simulink model "closed12augs"  (R2018b)
settings: Solver=VariableStepAuto  StartTime=0.0  StopTime=1  RelTol=1e-3
libraries: powerlib x63, simulink x5, autolibsharedcoupling x1, simulink_extras x1
settings Model: Creator=Ratish Kumar S  LastModifiedBy=Ratish Kumar S

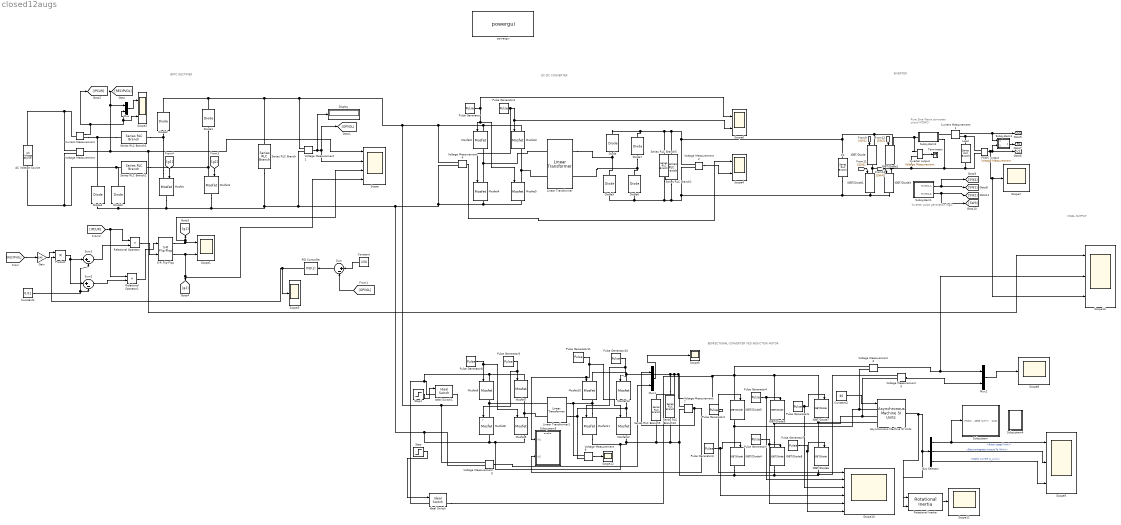
== system closed12augs ==
  note: INVERTER
  note: DC-DC CONVERTER
  note: Inverter pulse generation logic
  note: BPFC RECTIFIER
  note: Pure Sine Wave converter circuit (PSWC)
  note: z
  note: BIDIRECTIONAL CONVERTER FED INDUCTION MOTOR
  note: FINAL OUTPUT
  AC Voltage Source : powerlib/Electrical Sources/AC Voltage Source  Amplitude=230  Phase=0  Frequency=50  SampleTime=0  Measurements=None  BusType=swing  Pref=10e3  Qref=0  Qmin=-inf  Qmax=+inf
      settings: SourceProductName=Simscape Electrical
  Asynchronous Machine SI Units : powerlib/Machines/Asynchronous Machine SI Units  RotorType=Squirrel-cage  PresetModel=No  MechanicalLoad=Torque Tm  ShowDetailedParameters=on  ReferenceFrame=Rotor  Units=SI  MeasurementBus=off  NominalParameters=[1.845e+04 380 50]  Stator=[0.699999 0.00999999]  Rotor=[0.6258 0.005473]  Cage1=[0.4155 0.002066]  Cage2=[0.4168 0.0003495]  Lm=0.0399  Mechanical=[0.05 0.005879 2]  PolePairs=2  InitialConditions=[0 0 0 0 0 0 0 0]  SimulateSaturation=off  Saturation=[14.03593122, 27.81365428, 53.79336849, 72.68890987, 97.98006896, 148.6815601, 215.7428561, 302.9841135, 428.7778367 ; 230, 322, 414, 460, 506, 552, 598, 644, 690]  LoadFlowParameters=1492000  TsPowergui=0  TsBlock=-1  IterativeModel=Trapezoidal non iterative  IterativeDiscreteModel=Trapezoidal non iterative  Pmec=1.492e+006
      settings: SourceProductName=Simscape Electrical
  Bus Selector : BusSelector  OutputSignals=Mechanical.Rotor speed (wm),Mechanical.Electromagnetic torque Te (N*m),Stator measurements.Stator current is_a (A)
  C1 : powerlib/Elements/Series RLC Branch  LConnTagsString=__new0  RConnTagsString=__new0  BranchType=C  Resistance=1  Inductance=1e-3  SetiL0=off  InitialCurrent=0  Capacitance=200e-3  Setx0=off  InitialVoltage=0  Measurements=None
      settings: SourceProductName=Simscape Electrical
  Constant : Constant  Value=230
  Constant1 : Constant  Value=0.01
  Constant2 : Constant  Value=30
  Current Measurement : powerlib/Measurements/Current Measurement  PhasorSimulation=off  OutputType=Complex  PSBequivalent=0
      settings: SourceProductName=Simscape Electrical
  Current Measurement1 : powerlib/Measurements/Current Measurement  PhasorSimulation=off  OutputType=Complex  PSBequivalent=0
      settings: SourceProductName=Simscape Electrical
  Diode{,1..7} (8 alike) : powerlib/Power Electronics/Diode  Ron=0.001  Lon=0  Vf=0.8  IC=0  UseSnubber=off  Rs=500  Cs=250e-9  Measurements=off
      settings: SourceProductName=Simscape Electrical
  Display : Display
  Gain : Gain  Gain=1/40
  IGBT/Diode{,1..3} (4 alike) : powerlib/Power Electronics/IGBT//Diode  Ron=1e-3  Rs=1e5  Cs=inf  Measurements=off
      settings: SourceProductName=Simscape Electrical
  IGBT/Diode{4..9} (6 alike) : powerlib/Power Electronics/IGBT//Diode  Ron=1e-3  Rs=1e5  Cs=inf  Measurements=on
      settings: SourceProductName=Simscape Electrical
  Ideal Switch : powerlib/Power Electronics/Ideal Switch  Ron=0.001  Lon=0  IC=0  Rs=1e5  Cs=inf  Measurements=on
      settings: SourceProductName=Simscape Electrical
  Ideal Switch1 : powerlib/Power Electronics/Ideal Switch  Ron=0.001  Lon=0  IC=0  Rs=1e5  Cs=inf  Measurements=on
      settings: SourceProductName=Simscape Electrical
  Inverter output : powerlib/Measurements/Voltage Measurement  PhasorSimulation=off  OutputType=Complex  PSBequivalent=0
      settings: SourceProductName=Simscape Electrical
  Linear Transformer : powerlib/Elements/Linear Transformer  UNITS=SI  NominalPower=[5e3 50000 ]  winding1=[300 0.0004 0]  winding2=[170 0.0004 0]  ThreeWindings=off  winding3=[3.15e+05 24806 7.8961]  RmLm=[1000 21.518e-6]  Measurements=None  DataType=on
      settings: SourceProductName=Simscape Electrical
  Linear Transformer1 : powerlib/Elements/Linear Transformer  UNITS=SI  NominalPower=[8e3 20000 ]  winding1=[100 0.00025 0]  winding2=[100 0.0004 0]  ThreeWindings=off  winding3=[3.15e+05 24806 7.8961]  RmLm=[1000 360e-6]  Measurements=None  DataType=on
      settings: SourceProductName=Simscape Electrical
  Load : powerlib/Elements/Series RLC Branch  LConnTagsString=__new0  RConnTagsString=__new0  BranchType=R  Resistance=8  Inductance=10e-3  SetiL0=off  InitialCurrent=0  Capacitance=100e-6  Setx0=off  InitialVoltage=0  Measurements=None
      settings: SourceProductName=Simscape Electrical
  Mosfet : powerlib/Power Electronics/Mosfet  Ron=0.1  Lon=0  Rd=0.01  Vfd=0  IC=0  Rs=1e5  Cs=inf  Measurements=off
      settings: SourceProductName=Simscape Electrical
  Mosfet1 : powerlib/Power Electronics/Mosfet  Ron=0.1  Lon=0  Rd=0.01  Vfd=0  IC=0  Rs=1e5  Cs=inf  Measurements=off
      settings: SourceProductName=Simscape Electrical
  Mosfet{10..13} (4 alike) : powerlib/Power Electronics/Mosfet  Ron=5e-3  Lon=0  Rd=5e-3  Vfd=1  IC=0  Rs=1e5  Cs=inf  Measurements=on
      settings: SourceProductName=Simscape Electrical
  Mosfet{2..9} (8 alike) : powerlib/Power Electronics/Mosfet  Ron=2e-3  Lon=0  Rd=2e-3  Vfd=1  IC=0  Rs=1e5  Cs=inf  Measurements=on
      settings: SourceProductName=Simscape Electrical
  Mux : Mux  Inputs=2
  Mux1 : Mux  Inputs=2
  Mux2 : Mux  Inputs=2
  PID Controller : simulink/Continuous/PID Controller  Controller=PID  Form=Parallel  TimeDomain=Continuous-time  SampleTime=-1  IntegratorMethod=Forward Euler  FilterMethod=Forward Euler  ControllerParametersSource=internal  P=-0.01  I=1  D=7.5  UseFilter=on  N=1  TunerSelectOption=Transfer Function Based (PID Tuner App)  ZeroCross=off  InitialConditionSource=internal  InitialConditionForIntegrator=0  InitialConditionForFilter=0  DifferentiatorICPrevScaledInput=0  ExternalReset=none  TrackingMode=off  Kt=1  LimitOutput=off  UpperSaturationLimit=inf  LowerSaturationLimit=-inf  LinearizeAsGain=on  AntiWindupMode=none  Kb=1  POutMin=[]  POutMax=[]  IOutMin=[]  IOutMax=[]  DOutMin=[]  DOutMax=[]  NOutMin=[]  NOutMax=[]  SumOutMin=[]  SumOutMax=[]  SaturationOutMin=[]  SaturationOutMax=[]  PParamMin=[]  PParamMax=[]  IParamMin=[]  IParamMax=[]  DParamMin=[]  DParamMax=[]  NParamMin=[]  NParamMax=[]  KbParamMin=[]  KbParamMax=[]  KtParamMin=[]  KtParamMax=[]  KbOutMin=[]  KbOutMax=[]  KtOutMin=[]  KtOutMax=[]  IntegratorOutMin=[]  IntegratorOutMax=[]  FilterOutMin=[]  FilterOutMax=[]  SumI1OutMin=[]  SumI1OutMax=[]  SumI2OutMin=[]  SumI2OutMax=[]  SumI3OutMin=[]  SumI3OutMax=[]  SumI4OutMin=[]  SumI4OutMax=[]  SumDOutMin=[]  SumDOutMax=[]  DifferentiatorOutMin=[]  DifferentiatorOutMax=[]  FilterDiffOutCoefMin=[]  FilterDiffOutCoefMax=[]  ReciprocalOutMin=[]  ReciprocalOutMax=[]  SumDenOutMin=[]  SumDenOutMax=[]  SumNumOutMin=[]  SumNumOutMax=[]  DivideOutMin=[]  DivideOutMax=[]  IntegratorContinuousStateAttributes=''  IntegratorStateMustResolveToSignalObject=off  IntegratorRTWStateStorageClass=Auto  FilterContinuousStateAttributes=''  FilterStateMustResolveToSignalObject=off  FilterRTWStateStorageClass=Auto  ParallelPVariant=InternalParameters  IdealPVariant=Disabled  IVariant=InternalParameters  DVariant=InternalParameters  IntegratorVariant=Continuous  SatVariant=Disabled  AWVariant=Passthrough  PCopyVariant=Disabled  TRVariant=Disabled  FdbkBlocksVariant=Forward  IdealPFdbkVariant=Disabled  SatFdbkVariant=Disabled  DerivativeFilterVariant=ContFilter  NVariant=InternalParameters  NCopyVariant=Disabled  FilterICVariant=InternalICsFilter  IntegratorICVariant=InternalICs  ExternalResetVariant=Disabled  TRSumVariant=Passthrough  SumFdbkVariant=Disabled  SumVariant=Sum_PID
  PSWC output : powerlib/Measurements/Voltage Measurement  PhasorSimulation=off  OutputType=Complex  PSBequivalent=0
      settings: SourceProductName=Simscape Electrical
  Product : Product
  Pulse Generator : DiscretePulseGenerator  PulseType=Time based  Period=.00002  PulseWidth=50  VectorParams1D=off
  Pulse Generator1 : DiscretePulseGenerator  PulseType=Time based  Period=.00002  PulseWidth=50  PhaseDelay=2.22e-10  VectorParams1D=off
  Pulse Generator10 : DiscretePulseGenerator  PulseType=Time based  Amplitude=5  Period=50e-6  PulseWidth=50  PhaseDelay=25e-6
  Pulse Generator11 : DiscretePulseGenerator  PulseType=Time based  Amplitude=5  Period=50e-6  PulseWidth=50
  Pulse Generator2 : DiscretePulseGenerator  PulseType=Time based  Period=.02  PulseWidth=33
  Pulse Generator3 : DiscretePulseGenerator  PulseType=Time based  Period=.02  PulseWidth=33  PhaseDelay=.01
  Pulse Generator4 : DiscretePulseGenerator  PulseType=Time based  Period=.02  PulseWidth=33  PhaseDelay=.0066
  Pulse Generator5 : DiscretePulseGenerator  PulseType=Time based  Period=.02  PulseWidth=33  PhaseDelay=.0166
  Pulse Generator6 : DiscretePulseGenerator  PulseType=Time based  Period=.02  PulseWidth=33  PhaseDelay=.0133
  Pulse Generator7 : DiscretePulseGenerator  PulseType=Time based  Period=.02  PulseWidth=33  PhaseDelay=.0033
  Pulse Generator8 : DiscretePulseGenerator  PulseType=Time based  Amplitude=5  Period=50e-6  PulseWidth=50
  Pulse Generator9 : DiscretePulseGenerator  PulseType=Time based  Amplitude=5  Period=50e-6  PulseWidth=50  PhaseDelay=25e-6
  Relational Operator : RelationalOperator  Operator=>  OutDataTypeStr=boolean  RndMeth=Nearest
  Relational Operator1 : RelationalOperator  Operator=<  OutDataTypeStr=boolean  RndMeth=Nearest
  Rotational Inertia : autolibsharedcoupling/Rotational Inertia  port_config=Simulink  J=.01  b=.001  omega_o=0  externJ=off  blkID=0  aMode=2
      settings: SourceProductName=Powertrain Blockset  SourceProductBaseCode=PW
  S-R Flip-Flop : simulink_extras/Flip Flops/S-R Flip-Flop  initial_condition=0
  Scope : Scope  NumInputPorts=4
  Scope{1..2,4,6} (4 alike) : Scope  NumInputPorts=2
  Scope10 : Scope  NumInputPorts=6
  Scope{3,5,7..8,11..12} (6 alike) : Scope
  Scope13 : Scope  NumInputPorts=3
  Scope9 : Scope  NumInputPorts=3
  Series RLC Branch : powerlib/Elements/Series RLC Branch  LConnTagsString=__new0  RConnTagsString=__new0  BranchType=C  Resistance=1  Inductance=1e-3  SetiL0=off  InitialCurrent=0  Capacitance=100e-6  Setx0=off  InitialVoltage=0  Measurements=None
      settings: SourceProductName=Simscape Electrical
  Series RLC Branch1 : powerlib/Elements/Series RLC Branch  LConnTagsString=__new0  RConnTagsString=__new0  BranchType=R  Resistance=100  Inductance=1e-3  SetiL0=off  InitialCurrent=0  Capacitance=1e-6  Setx0=off  InitialVoltage=0  Measurements=None
      settings: SourceProductName=Simscape Electrical
  Series RLC Branch10 : powerlib/Elements/Series RLC Branch  LConnTagsString=__new0  RConnTagsString=__new0  BranchType=R  Resistance=15  Inductance=1e-3  SetiL0=off  InitialCurrent=0  Capacitance=10e-6  Setx0=off  InitialVoltage=0  Measurements=Branch voltage
      settings: SourceProductName=Simscape Electrical
  Series RLC Branch2 : powerlib/Elements/Series RLC Branch  LConnTagsString=__new0  RConnTagsString=__new0  BranchType=L  Resistance=1  Inductance=5e-3  SetiL0=off  InitialCurrent=0  Capacitance=1e-6  Setx0=off  InitialVoltage=0  Measurements=None
      settings: SourceProductName=Simscape Electrical
  Series RLC Branch3 : powerlib/Elements/Series RLC Branch  LConnTagsString=__new0  RConnTagsString=__new0  BranchType=L  Resistance=1  Inductance=5e-3  SetiL0=off  InitialCurrent=0  Capacitance=1e-6  Setx0=off  InitialVoltage=0  Measurements=None
      settings: SourceProductName=Simscape Electrical
  Series RLC Branch5 : powerlib/Elements/Series RLC Branch  LConnTagsString=__new0  RConnTagsString=__new0  BranchType=C  Resistance=1  Inductance=1e-3  SetiL0=off  InitialCurrent=0  Capacitance=300e-5  Setx0=off  InitialVoltage=0  Measurements=Branch voltage
      settings: SourceProductName=Simscape Electrical
  Series RLC Branch9 : powerlib/Elements/Series RLC Branch  LConnTagsString=__new0  RConnTagsString=__new0  BranchType=C  Resistance=1  Inductance=1e-3  SetiL0=off  InitialCurrent=0  Capacitance=10000e-6  Setx0=off  InitialVoltage=0  Measurements=Branch voltage
      settings: SourceProductName=Simscape Electrical
  Step : Step  Time=0.05  SampleTime=0
  Step1 : Step  Time=0.05  Before=1  After=0  SampleTime=0
  Subsystem : Subsystem
  Subsystem1 : Subsystem
  Subsystem2 : Subsystem
  Subsystem3 : Subsystem
  Subsystem4 : Subsystem
  Subsystem5 : Subsystem
  Sum : Sum  Inputs=|+-
  Sum1 : Sum  Inputs=|+-
  Sum2 : Sum  Inputs=|+-
  Terminator : Terminator
  Voltage Measurement{,1..5,7..9} (9 alike) : powerlib/Measurements/Voltage Measurement  PhasorSimulation=off  OutputType=Complex  PSBequivalent=0
      Voltage Measurement settings: SourceProductName=Simscape Electrical
      Voltage Measurement1 settings: SourceProductName=Simscape Electrical
      Voltage Measurement2 settings: SourceProductName=Simscape Electrical
      Voltage Measurement4 settings: SourceProductName=Simscape Electrical
      Voltage Measurement7 settings: SourceProductName=Simscape Electrical
      Voltage Measurement8 settings: SourceProductName=Simscape Electrical
      Voltage Measurement9 settings: SourceProductName=Simscape Electrical
  powergui : powerlib/powergui  Priority=1  SimulationMode=Discrete  SampleTime=1e-6  frequency=60  Iterations=50  frequencyindice=0  Pbase=100e6  ErrMax=1e-4  UnitsV=kV  UnitsW=MW  buscounter=0  FunctionMessages=off  echomessages=off  EnableUseOfTLC=off  CurrentSourceSwitches=off  DisableSnubberDevices=off  DisableRonSwitches=off  DisableVfSwitches=off  DisplayEquations=off  SolverType=Tustin/Backward Euler (TBE)  Interpol=off  ExternalGateDelay=off  methode=off  Ts=100  x0status=blocks  SPID=off  SwTol=0  HookPort=off  RestoreLinks=warning  ResistiveCurrentMeasurement=off  Frange=[0:2:500]  Ylog=off  Xlog=on  ShowGrid=off  save=off  variable=ZData  structure=0  ZoomFFT=off  StartTime=0.0  cycles=1  DisplayStyle=1  fundamental=60  FreqAxis=off  MaxFrequency=1000  frequencyindicesteady=1  RmsSteady=1  display=off
  wires:
  Current Measurement1/1 -> Subsystem3/1(In1), [I2]
  Subsystem3/1(Out1) -> [P2]
  Subsystem1/2(To SW2,3) -> [SW3], [SW2]
  [SW1] -> IGBT/Diode/1
  [SW4] -> IGBT/Diode3/1
  [SW2] -> IGBT/Diode2/1
  Inverter output/1 -> Terminator/1
  [SW3] -> IGBT/Diode1/1
  Mux/1 -> Scope2/1
  S-R Flip-Flop/2 -> [g2], Scope/4, Scope1/2
  Pulse Generator1/1 -> Scope6/2, Mosfet3/1, Mosfet4/1
  PSWC output/1 -> Scope13/3, Scope7/1, [V2], Subsystem3/2(In2)
  Pulse Generator/1 -> Scope6/1, Mosfet2/1, Mosfet5/1
  Voltage Measurement4/1 -> Scope4/1
  Relational Operator/1 -> S-R Flip-Flop/2
  [OPVOL] -> Sum/2
  Voltage Measurement1/1 -> Display/1, [OPVOL], Scope/2
  Constant1/1 -> Sum1/2, Sum2/2
  PID Controller/1 -> Scope3/1, Product/2
  Voltage Measurement2/1 -> Scope4/2
  Relational Operator1/1 -> S-R Flip-Flop/1
  [g2] -> Mosfet1/1
  Sum2/1 -> Relational Operator1/2
  Sum1/1 -> Relational Operator/2
  [IPCUR] -> Relational Operator1/1, Relational Operator/1
  Subsystem1/1(To SW1,4) -> [SW1], [SW4]
  Voltage Measurement/1 -> Scope13/1, Scope/1, [RECIPVOL], Mux/1
  [RECIPVOL] -> Gain/1
  Gain/1 -> Product/1
  S-R Flip-Flop/1 -> Scope/3, [g1], Scope1/1
  Current Measurement/1 -> Scope2/2, Mux/2, [IPCUR]
  Constant/1 -> Sum/1
  Sum/1 -> PID Controller/1
  [g1] -> Mosfet/1
  Product/1 -> Sum2/1, Sum1/1
  Pulse Generator7/1 -> Scope10/6, IGBT/Diode6/1
  Step1/1 -> Ideal Switch1/1
  Pulse Generator4/1 -> Scope10/2, IGBT/Diode9/1
  Pulse Generator5/1 -> Scope10/5, IGBT/Diode8/1
  Voltage Measurement8/1 -> Scope12/1
  Step/1 -> Ideal Switch/1
  Voltage Measurement9/1 -> Mux1/2
  Bus Selector/1 -> Subsystem/1(<Rotor speed (wm)>), Scope9/1  "<Rotor speed (wm)>"
  Pulse Generator6/1 -> Scope10/3, IGBT/Diode7/1
  Pulse Generator9/1 -> Mosfet8/1, Mosfet7/1
  Constant2/1 -> Asynchronous Machine SI Units/1
  Bus Selector/3 -> Scope9/3  "<Stator current is_a (A)>"
  Asynchronous Machine SI Units/1 -> Rotational Inertia/1, Rotational Inertia/2, Bus Selector/1
  Rotational Inertia/1 -> Scope11/1
  Pulse Generator3/1 -> Scope10/4, IGBT/Diode4/1
  Voltage Measurement7/1 -> Mux1/1, Subsystem5/2(In2)
  Pulse Generator2/1 -> Scope10/1, IGBT/Diode5/1
  Mux1/1 -> Scope5/1
  Pulse Generator8/1 -> Mosfet6/1, Mosfet9/1
  Pulse Generator10/1 -> Mosfet11/1, Mosfet13/1
  Pulse Generator11/1 -> Subsystem5/1(In1), Mosfet10/1, Mosfet12/1
  Bus Selector/2 -> Scope9/2  "<Electromagnetic torque Te (N*m)>"
  Voltage Measurement5/1 -> Mux2/2
  Voltage Measurement3/1 -> Scope13/2, Mux2/1
  Mux2/1 -> Scope8/1
  connections:
  Current Measurement1/RConn1 -- Load/LConn1 -- PSWC output/LConn1
  IGBT/Diode2/RConn1 -- IGBT/Diode3/LConn1 -- Inverter output/LConn2 -- Subsystem2/RConn2 -- Load/RConn1 -- PSWC output/LConn2
  Inverter output/LConn1 -- Subsystem2/LConn1 -- IGBT/Diode1/LConn1 -- IGBT/Diode/RConn1
  Diode5/LConn1 -- Diode6/LConn1 -- Series RLC Branch5/RConn1 -- Voltage Measurement2/LConn2 -- C1/RConn1 -- IGBT/Diode3/RConn1 -- IGBT/Diode1/RConn1 -- Series RLC Branch1/RConn1
  Diode5/RConn1 -- Linear Transformer/RConn1 -- Diode/LConn1
  Diode7/RConn1 -- Series RLC Branch5/LConn1 -- IGBT/Diode/LConn1 -- IGBT/Diode2/LConn1 -- C1/LConn1 -- Voltage Measurement2/LConn1 -- Series RLC Branch1/LConn1 -- Diode/RConn1
  Series RLC Branch9/RConn1 -- Voltage Measurement9/LConn2 -- Mosfet5/RConn1 -- Mosfet4/RConn1 -- Voltage Measurement4/LConn2 -- Voltage Measurement1/LConn2 -- Series RLC Branch/RConn1 -- Mosfet1/RConn1 -- Diode3/LConn1 -- Diode4/LConn1 -- Mosfet/RConn1 -- Mosfet8/RConn1 -- Mosfet9/RConn1 -- Mosfet11/RConn1 -- Mosfet12/RConn1 -- Series RLC Branch10/RConn1 -- IGBT/Diode4/RConn1 -- IGBT/Diode8/RConn1 -- Voltage Measurement5/LConn1 -- IGBT/Diode6/RConn1 -- Voltage Measurement7/LConn2
  Mosfet3/RConn1 -- Linear Transformer/LConn2 -- Mosfet5/LConn1
  Linear Transformer/RConn2 -- Diode6/RConn1 -- Diode7/LConn1
  Mosfet/LConn1 -- Diode2/LConn1 -- Series RLC Branch3/RConn1
  Ideal Switch1/RConn1 -- Voltage Measurement9/LConn1 -- Voltage Measurement4/LConn1 -- Mosfet3/LConn1 -- Mosfet2/LConn1 -- Series RLC Branch/LConn1 -- Diode2/RConn1 -- Diode1/RConn1 -- Voltage Measurement1/LConn1
  Mosfet2/RConn1 -- Linear Transformer/LConn1 -- Mosfet4/LConn1
  AC Voltage Source/LConn1 -- Voltage Measurement/LConn2 -- Diode3/RConn1 -- Series RLC Branch2/LConn1
  Series RLC Branch3/LConn1 -- Diode4/RConn1 -- Current Measurement/RConn1
  AC Voltage Source/RConn1 -- Voltage Measurement/LConn1 -- Current Measurement/LConn1
  Mosfet1/LConn1 -- Series RLC Branch2/RConn1 -- Diode1/LConn1
  Current Measurement1/LConn1 -- Subsystem2/RConn1
  Mosfet12/LConn1 -- Mosfet13/RConn1 -- Voltage Measurement8/LConn2 -- Linear Transformer1/RConn2
  Ideal Switch/LConn1 -- Ideal Switch1/LConn1 -- Mosfet6/LConn1 -- Mosfet7/LConn1
  Series RLC Branch10/LConn1 -- Mosfet10/LConn1 -- Mosfet13/LConn1 -- Ideal Switch/RConn1 -- IGBT/Diode5/LConn1 -- Voltage Measurement3/LConn1 -- IGBT/Diode9/LConn1 -- IGBT/Diode7/LConn1 -- Voltage Measurement7/LConn1 -- Series RLC Branch9/LConn1
  Mosfet7/RConn1 -- Linear Transformer1/LConn2 -- Mosfet9/LConn1
  Mosfet11/LConn1 -- Voltage Measurement8/LConn1 -- Linear Transformer1/RConn1 -- Mosfet10/RConn1
  Mosfet8/LConn1 -- Linear Transformer1/LConn1 -- Mosfet6/RConn1
  IGBT/Diode8/LConn1 -- Voltage Measurement5/LConn2 -- Asynchronous Machine SI Units/LConn2 -- IGBT/Diode9/RConn1
  IGBT/Diode4/LConn1 -- Voltage Measurement3/LConn2 -- Asynchronous Machine SI Units/LConn1 -- IGBT/Diode5/RConn1
  Asynchronous Machine SI Units/LConn3 -- IGBT/Diode6/LConn1 -- IGBT/Diode7/RConn1

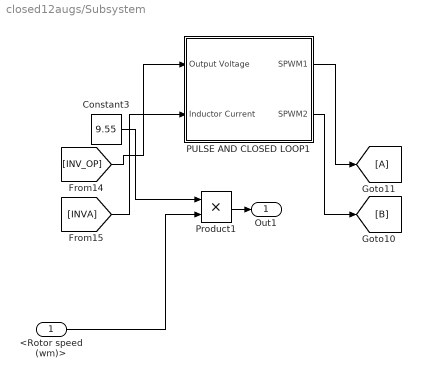
== system closed12augs/Subsystem ==
  <Rotor speed (wm)> : Inport
  Constant3 : Constant  Value=9.55
  PULSE AND CLOSED LOOP1 : Subsystem
  Product1 : Product
  Out1 : Outport
  wires:
  <Rotor speed (wm)>/1 -> Product1/2
  [INV_OP] -> PULSE AND CLOSED LOOP1/1("Output Voltage ")
  PULSE AND CLOSED LOOP1/1(SPWM1) -> [A]
  PULSE AND CLOSED LOOP1/2(SPWM2) -> [B]
  [INVA] -> PULSE AND CLOSED LOOP1/2(Inductor Current)
  Constant3/1 -> Product1/1
  Product1/1 -> Out1/1

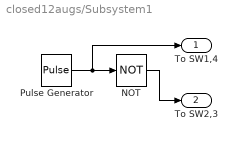
== system closed12augs/Subsystem1 ==
  NOT : Logic  Operator=NOT  IconShape=distinctive  AllPortsSameDT=off  OutDataTypeStr=boolean
  Pulse Generator : DiscretePulseGenerator  PulseType=Time based  Period=1/50  PulseWidth=50
  To SW1,4 : Outport
  To SW2,3 : Outport  Port=2
  wires:
  NOT/1 -> To SW2,3/1
  Pulse Generator/1 -> To SW1,4/1, NOT/1

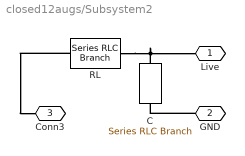
== system closed12augs/Subsystem2 ==
  C : powerlib/Elements/Series RLC Branch  LConnTagsString=__new0  RConnTagsString=__new0  BranchType=C  Resistance=1  Inductance=1e-3  SetiL0=off  InitialCurrent=0  Capacitance=300e-6  Setx0=off  InitialVoltage=0  Measurements=None
      settings: SourceProductName=Simscape Electrical
  RL : powerlib/Elements/Series RLC Branch  LConnTagsString=__new0  RConnTagsString=__new0  BranchType=RL  Resistance=1.25  Inductance=40e-3  SetiL0=off  InitialCurrent=0  Capacitance=1000e-6  Setx0=off  InitialVoltage=0  Measurements=None
      settings: SourceProductName=Simscape Electrical
  Live : PMIOPort  Side=Right
  GND : PMIOPort  Port=2  Side=Right
  Conn3 : PMIOPort  Port=3  Side=Left
  connections:
  GND/RConn1 -- C/RConn1
  RL/LConn1 -- Conn3/RConn1
  C/LConn1 -- Live/RConn1 -- RL/RConn1

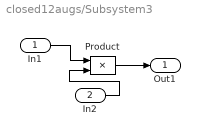
== system closed12augs/Subsystem3 ==
  In1 : Inport
  In2 : Inport  Port=2
  Product : Product
  Out1 : Outport
  wires:
  In2/1 -> Product/2
  In1/1 -> Product/1
  Product/1 -> Out1/1

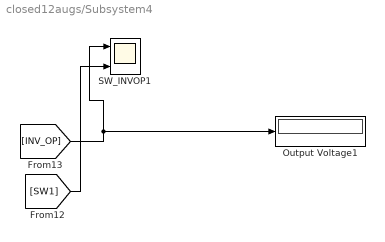
== system closed12augs/Subsystem4 ==
  Output Voltage1 : Display
  SW_INVOP1 : Scope  NumInputPorts=2
  wires:
  [SW1] -> SW_INVOP1/2
  [INV_OP] -> Output Voltage1/1, SW_INVOP1/1

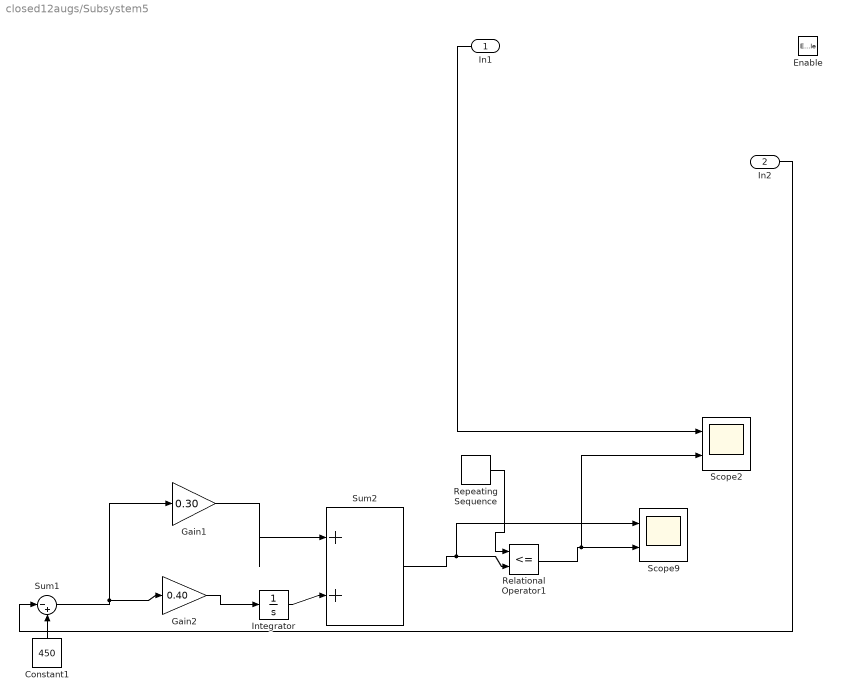
== system closed12augs/Subsystem5 ==
  In1 : Inport
  In2 : Inport  Port=2
  Enable : EnablePort
  Constant1 : Constant  Value=450
  Gain1 : Gain  Gain=0.30
  Gain2 : Gain  Gain=0.40
  Integrator : Integrator
  Relational Operator1 : RelationalOperator  Operator=<=  OutDataTypeStr=boolean  RndMeth=Nearest
  Repeating Sequence : simulink/Sources/Repeating Sequence  rep_seq_t=[0 20e-6]  rep_seq_y=[0 15]
  Scope2 : Scope  NumInputPorts=2
  Scope9 : Scope  NumInputPorts=2
  Sum1 : Sum  Inputs=|-+
  Sum2 : Sum  Inputs=|++
  wires:
  Sum2/1 -> Relational Operator1/2, Scope9/1
  Gain2/1 -> Integrator/1
  Integrator/1 -> Sum2/2
  Relational Operator1/1 -> Scope9/2, Scope2/2
  Repeating Sequence/1 -> Relational Operator1/1
  Gain1/1 -> Sum2/1
  Sum1/1 -> Gain1/1, Gain2/1
  In2/1 -> Sum1/1
  Constant1/1 -> Sum1/2
  In1/1 -> Scope2/1

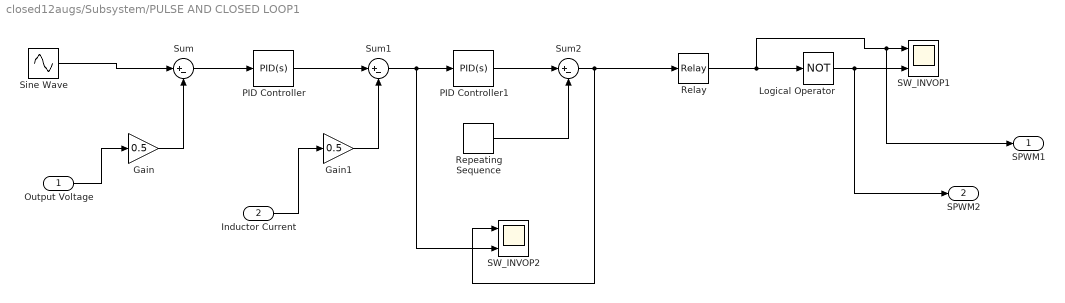
== system closed12augs/Subsystem/PULSE AND CLOSED LOOP1 ==
  "Output Voltage " : Inport
  Inductor Current : Inport  Port=2
  Gain : Gain  Gain=0.5
  Gain1 : Gain  Gain=0.5
  Logical Operator : Logic  Operator=NOT  AllPortsSameDT=off  OutDataTypeStr=boolean
  PID Controller : simulink/Continuous/PID Controller  Controller=PID  Form=Parallel  TimeDomain=Continuous-time  SampleTime=-1  IntegratorMethod=Forward Euler  FilterMethod=Forward Euler  ControllerParametersSource=internal  P=-29179196.3770785  I=-660.576216727273  D=-244938248740.003  UseFilter=on  N=0.106241712953446  TunerSelectOption=Transfer Function Based (PID Tuner App)  InitialConditionSource=internal  InitialConditionForIntegrator=0  InitialConditionForFilter=0  DifferentiatorICPrevScaledInput=0  ExternalReset=none  TrackingMode=off  Kt=1  LimitOutput=off  UpperSaturationLimit=inf  LowerSaturationLimit=-inf  LinearizeAsGain=on  AntiWindupMode=none  Kb=1  POutMin=[]  POutMax=[]  IOutMin=[]  IOutMax=[]  DOutMin=[]  DOutMax=[]  NOutMin=[]  NOutMax=[]  SumOutMin=[]  SumOutMax=[]  SaturationOutMin=[]  SaturationOutMax=[]  PParamMin=[]  PParamMax=[]  IParamMin=[]  IParamMax=[]  DParamMin=[]  DParamMax=[]  NParamMin=[]  NParamMax=[]  KbParamMin=[]  KbParamMax=[]  KtParamMin=[]  KtParamMax=[]  KbOutMin=[]  KbOutMax=[]  KtOutMin=[]  KtOutMax=[]  IntegratorOutMin=[]  IntegratorOutMax=[]  FilterOutMin=[]  FilterOutMax=[]  SumI1OutMin=[]  SumI1OutMax=[]  SumI2OutMin=[]  SumI2OutMax=[]  SumI3OutMin=[]  SumI3OutMax=[]  SumI4OutMin=[]  SumI4OutMax=[]  SumDOutMin=[]  SumDOutMax=[]  DifferentiatorOutMin=[]  DifferentiatorOutMax=[]  FilterDiffOutCoefMin=[]  FilterDiffOutCoefMax=[]  ReciprocalOutMin=[]  ReciprocalOutMax=[]  SumDenOutMin=[]  SumDenOutMax=[]  SumNumOutMin=[]  SumNumOutMax=[]  DivideOutMin=[]  DivideOutMax=[]  IntegratorContinuousStateAttributes=''  IntegratorStateMustResolveToSignalObject=off  IntegratorRTWStateStorageClass=Auto  FilterContinuousStateAttributes=''  FilterStateMustResolveToSignalObject=off  FilterRTWStateStorageClass=Auto  ParallelPVariant=InternalParameters  IdealPVariant=Disabled  IVariant=InternalParameters  DVariant=InternalParameters  IntegratorVariant=Continuous  SatVariant=Disabled  AWVariant=Passthrough  PCopyVariant=Disabled  TRVariant=Disabled  FdbkBlocksVariant=Forward  IdealPFdbkVariant=Disabled  SatFdbkVariant=Disabled  DerivativeFilterVariant=ContFilter  NVariant=InternalParameters  NCopyVariant=Disabled  FilterICVariant=InternalICsFilter  IntegratorICVariant=InternalICs  ExternalResetVariant=Disabled  TRSumVariant=Passthrough  SumFdbkVariant=Disabled  SumVariant=Sum_PID
  PID Controller1 : simulink/Continuous/PID Controller  Controller=PID  Form=Parallel  TimeDomain=Continuous-time  SampleTime=-1  IntegratorMethod=Forward Euler  FilterMethod=Forward Euler  ControllerParametersSource=internal  P=4.19313609887985e-16  I=2.36776520880665e-19  D=7.14204463612493e-14  UseFilter=on  N=1.02395165861612  TunerSelectOption=Transfer Function Based (PID Tuner App)  InitialConditionSource=internal  InitialConditionForIntegrator=0  InitialConditionForFilter=0  DifferentiatorICPrevScaledInput=0  ExternalReset=none  TrackingMode=off  Kt=1  LimitOutput=off  UpperSaturationLimit=inf  LowerSaturationLimit=-inf  LinearizeAsGain=on  AntiWindupMode=none  Kb=1  POutMin=[]  POutMax=[]  IOutMin=[]  IOutMax=[]  DOutMin=[]  DOutMax=[]  NOutMin=[]  NOutMax=[]  SumOutMin=[]  SumOutMax=[]  SaturationOutMin=[]  SaturationOutMax=[]  PParamMin=[]  PParamMax=[]  IParamMin=[]  IParamMax=[]  DParamMin=[]  DParamMax=[]  NParamMin=[]  NParamMax=[]  KbParamMin=[]  KbParamMax=[]  KtParamMin=[]  KtParamMax=[]  KbOutMin=[]  KbOutMax=[]  KtOutMin=[]  KtOutMax=[]  IntegratorOutMin=[]  IntegratorOutMax=[]  FilterOutMin=[]  FilterOutMax=[]  SumI1OutMin=[]  SumI1OutMax=[]  SumI2OutMin=[]  SumI2OutMax=[]  SumI3OutMin=[]  SumI3OutMax=[]  SumI4OutMin=[]  SumI4OutMax=[]  SumDOutMin=[]  SumDOutMax=[]  DifferentiatorOutMin=[]  DifferentiatorOutMax=[]  FilterDiffOutCoefMin=[]  FilterDiffOutCoefMax=[]  ReciprocalOutMin=[]  ReciprocalOutMax=[]  SumDenOutMin=[]  SumDenOutMax=[]  SumNumOutMin=[]  SumNumOutMax=[]  DivideOutMin=[]  DivideOutMax=[]  IntegratorContinuousStateAttributes=''  IntegratorStateMustResolveToSignalObject=off  IntegratorRTWStateStorageClass=Auto  FilterContinuousStateAttributes=''  FilterStateMustResolveToSignalObject=off  FilterRTWStateStorageClass=Auto  ParallelPVariant=InternalParameters  IdealPVariant=Disabled  IVariant=InternalParameters  DVariant=InternalParameters  IntegratorVariant=Continuous  SatVariant=Disabled  AWVariant=Passthrough  PCopyVariant=Disabled  TRVariant=Disabled  FdbkBlocksVariant=Forward  IdealPFdbkVariant=Disabled  SatFdbkVariant=Disabled  DerivativeFilterVariant=ContFilter  NVariant=InternalParameters  NCopyVariant=Disabled  FilterICVariant=InternalICsFilter  IntegratorICVariant=InternalICs  ExternalResetVariant=Disabled  TRSumVariant=Passthrough  SumFdbkVariant=Disabled  SumVariant=Sum_PID
  Relay : Relay
  Repeating Sequence : simulink/Sources/Repeating Sequence  rep_seq_t=[0 0.5 1]*(1/500)  rep_seq_y=[0 1 0]
  SW_INVOP1 : Scope  NumInputPorts=2
  SW_INVOP2 : Scope  NumInputPorts=2
  Sine Wave : Sin  Amplitude=130  Frequency=2*pi*50  SampleTime=0
  Sum : Sum  Inputs=|+-
  Sum1 : Sum  Inputs=|+-
  Sum2 : Sum  Inputs=|+-
  SPWM1 : Outport
  SPWM2 : Outport  Port=2
  wires:
  Repeating Sequence/1 -> Sum2/2
  Sum2/1 -> Relay/1, SW_INVOP2/1
  Logical Operator/1 -> SPWM2/1, SW_INVOP1/2
  Sine Wave/1 -> Sum/1
  Sum1/1 -> SW_INVOP2/2, PID Controller1/1
  Gain/1 -> Sum/2
  PID Controller1/1 -> Sum2/1
  PID Controller/1 -> Sum1/1
  Sum/1 -> PID Controller/1
  Gain1/1 -> Sum1/2
  Relay/1 -> Logical Operator/1, SPWM1/1, SW_INVOP1/1
  "Output Voltage "/1 -> Gain/1
  Inductor Current/1 -> Gain1/1
